simulink model "astron_hw_test_au50_64k_8in"  (R2021a)
settings: Solver=VariableStepDiscrete  StartTime=0.0  StopTime=32000  RelTol=1e-3
undefined symbols (not defined in the file): d0, d1, d2, d3, d4, d5, d6, d7, FFT, sr, Wideband_FFT
libraries: xbsIndex_r4 x1247, casper_library_misc x6, xps_library x1
(part 6 of 26)

== system astron_hw_test_au50_64k_8in/bram_in3 ==
  addr : Inport
  data_in : Inport  Port=2
  we : Inport  Port=3
  Terminator : Terminator
  Terminator1 : Terminator
  Terminator2 : Terminator
  astron_hw_test_au50_64k_8in_bram_in3_addr : xbsIndex_r4/Gateway Out  inherit_from_input=off  hdl_port=on  rows=1  columns=1  UseAsDAC=off  DACChannel='1'  interface=None  automatic_assignment=on  address_offset=hex2dec('00')  intf_name=''  intf_description=''  timing_constraint=None  locs_specified=off  LOCs={'A5','B9','A9','C1','A3','G6','E9','A6','A7','A8','B8','B1','B3','D9','B5','B4','B6','C2'}  io_standard={}  block_type=gatewayout
      settings: infoedit="Gateway out block.  Converts Xilinx fixed point inputs into ouputs of type Simulink integer, double, or fixed point.<P><P>Hardware notes:  In hardware these blocks become top level output ports or are discarded, depending on how they are configured."  sginterface={'Nallatech'=>{'xdspkit'=>{'non_memory_mapped_port'=>'uprev_Shared_BRAM_addr'}},'Xilinx'=>{'jtaghwcosim'=>{'non_memory_mapped_port'=>'uprev_Shared_BRAM_addr'},'xdspkit'=>{'non_memory_mapped_port'=>'uprev_Shared_BRAM_addr'}}}  xl_area=[0, 0, 0, 0, 0, 0, 0]
  astron_hw_test_au50_64k_8in_bram_in3_data_in : xbsIndex_r4/Gateway Out  inherit_from_input=off  hdl_port=on  rows=1  columns=1  UseAsDAC=off  DACChannel='1'  interface=None  automatic_assignment=on  address_offset=hex2dec('00')  intf_name=''  intf_description=''  timing_constraint=None  locs_specified=off  LOCs={'B21','B22','A22','B23','B19','C19','A20','A21','A23','B24','A24','A25','E18','D18','C18','B18'}  io_standard={}  block_type=gatewayout
      settings: infoedit="Gateway out block.  Converts Xilinx fixed point inputs into ouputs of type Simulink integer, double, or fixed point.<P><P>Hardware notes:  In hardware these blocks become top level output ports or are discarded, depending on how they are configured."  sginterface={'Nallatech'=>{'xdspkit'=>{'non_memory_mapped_port'=>'uprev_Shared_BRAM_data_in'}},'Xilinx'=>{'jtaghwcosim'=>{'non_memory_mapped_port'=>'uprev_Shared_BRAM_data_in'},'xdspkit'=>{'non_memory_mapped_port'=>'uprev_Shared_BRAM_data_in'}}}  xl_area=[0, 0, 0, 0, 0, 0, 0]
  astron_hw_test_au50_64k_8in_bram_in3_data_out : xbsIndex_r4/Gateway In  gui_display_data_type=Fixed-point  arith_type=Unsigned  n_bits=32  bin_pt=0  preci_type=Single  exp_width=8  frac_width=24  rows=1  columns=1  quantization=Truncate  overflow=Wrap  period=sample_rate  UseAsADC=off  ADCChannel='1'  interface=None  automatic_assignment=on  address_offset=hex2dec('00')  intf_name=''  intf_description=''  default_value=0  timing_constraint=None  locs_specified=off  LOCs={}  io_standard={}  inherit_from_input=off  hdl_port=on  dbl_ovrd=off  block_type=gatewayin
      settings: xl_area=[0, 0, 0, 0, 0, 0, 0]
  astron_hw_test_au50_64k_8in_bram_in3_we : xbsIndex_r4/Gateway Out  inherit_from_input=off  hdl_port=on  rows=1  columns=1  UseAsDAC=off  DACChannel='1'  interface=None  automatic_assignment=on  address_offset=hex2dec('00')  intf_name=''  intf_description=''  timing_constraint=None  locs_specified=off  LOCs={'A14'}  io_standard={}  block_type=gatewayout
      settings: infoedit="Gateway out block.  Converts Xilinx fixed point inputs into ouputs of type Simulink integer, double, or fixed point.<P><P>Hardware notes:  In hardware these blocks become top level output ports or are discarded, depending on how they are configured."  xl_area=[0, 0, 0, 0, 0, 0, 0]
  calc_add : Subsystem  mask{data_width=32, addr_width=13, sample_rate=sample_rate}
      mask prompts: data_width "data width"; addr_width "address width"; sample_rate "sample rate"
  convert_addr : xbsIndex_r4/Convert  gui_display_data_type=Fixed-point  arith_type=Unsigned  n_bits=addr_width  bin_pt=0  float_type=Single  exp_bits=8  fraction_bits=24  quantization=Truncate  overflow=Wrap  en=off  latency=0  pipeline=off  dbl_ovrd=off  block_type=convert
      settings: xl_area=[0, 0, 0, 0, 0, 0, 0]
  convert_din1 : xbsIndex_r4/Convert  gui_display_data_type=Fixed-point  arith_type=Unsigned  n_bits=32  bin_pt=0  float_type=Single  exp_bits=8  fraction_bits=24  quantization=Truncate  overflow=Wrap  en=off  latency=0  pipeline=off  dbl_ovrd=off  block_type=convert
      settings: xl_area=[0, 0, 0, 0, 0, 0, 0]
  convert_we : xbsIndex_r4/Convert  gui_display_data_type=Fixed-point  arith_type=Unsigned  n_bits=1  bin_pt=0  float_type=Single  exp_bits=8  fraction_bits=24  quantization=Truncate  overflow=Wrap  en=off  latency=0  pipeline=off  dbl_ovrd=off  block_type=convert
      settings: xl_area=[0, 0, 0, 0, 0, 0, 0]
  munge_in : Subsystem  AncestorBlock=casper_library_flow_control/munge  mask(munge){divisions=1, div_size=32, order=[0], arith_type_out=Unsigned, bin_pt_out=0}
      mask prompts: divisions "Number of divisions"; div_size "Division size (bits)"; order "Division packing order"; arith_type_out "Output arithmetic type"; bin_pt_out "Output binary point"
      mask help: Splits an input bus into the specified number of divisions and then recombines them in the order specified (most significant division = 0,least = number divisions-1)
      mask init:
      | munge_init(gcb, ...
      |     'divisions', divisions, ...
      |     'div_size', div_size, ...
      |     'order', order, ...
      |     'arith_type_out', arith_type_out, ...
      |     'bin_pt_out', bin_pt_out);
      settings: AttributesFormatString=|
      | split:32
      | join:0
      | Unsigned [32,0]
      mask TypeOptions arith_type_out: Unsigned | Signed  (2's comp) | Floating-point
  munge_out : Subsystem  AncestorBlock=casper_library_flow_control/munge  mask(munge){divisions=1, div_size=32, order=[0], arith_type_out=Signed  (2's comp), bin_pt_out=0}
      mask prompts: divisions "Number of divisions"; div_size "Division size (bits)"; order "Division packing order"; arith_type_out "Output arithmetic type"; bin_pt_out "Output binary point"
      mask help: Splits an input bus into the specified number of divisions and then recombines them in the order specified (most significant division = 0,least = number divisions-1)
      mask init:
      | munge_init(gcb, ...
      |     'divisions', divisions, ...
      |     'div_size', div_size, ...
      |     'order', order, ...
      |     'arith_type_out', arith_type_out, ...
      |     'bin_pt_out', bin_pt_out);
      settings: AttributesFormatString=|
      | split:32
      | join:0
      | Signed  (2's comp) [32,0]
      mask TypeOptions arith_type_out: Unsigned | Signed  (2's comp) | Floating-point
  sim_mem : Subsystem  mask{arith_type=Signed  (2's comp), addr_width=13, data_width=32, data_bin_pt=0, init_vals=[9831  -6047   1111  -1845    944    479  -1311  -4696  10466   2542   1296  -5528   5032   9085  -9007   3196   1045  -2612   4431   2747    701  -2394   4649   7953   7611  -2438    653  -7011   6485  -8623   2524  -5311   5832   3592   -951  -3611   -666  -3316    239  -2256  -3089   3750  -4638   2874   3427  -1997   9115   1935   4089 -10713   4822   2154    279   5735   6850   -832   -441  -4702  -6341    514   3095   -604   4622    495   7543  -1649   5852  -3513  -1426   5023   3080   5056  12109   2829    -89  -1958  -1635   -882   8086   4095   5011  -5808    892  -5959   3390   3640   4469   5622    600  -6979   -735  -1172   3021  -2489    -10 -10282  -7018 -14437   3342    918   4893  -8173   4321   8999   1488  -7407   5292  -5466   8451   -385   1054   1231   9655  -6940  -2235  -3834   2601  -2170   5686  -1603   5214   3496   2809   3538     95  -3789   1812   -759   6389   5558   3719  -1679  -3442   3537   1698  -5286    545    375   2542  -2227   3925   2425   1058   5149   5431   -340    165  -8569   3002  -7189   2921   7702  10866   1098   2719  -6821   5714   2275  -2093  -2390   3583   1045   3029  -5013   2806   4201   -826   4473   1926   3197   2662  -5326   -132  -7657   6141  -3966   1085   4296   2972     60   2145   3502    -45   -413   -959  -8354   5105  -1323 -10075  -3461   4303  -2691   2921   2691   2602  -4447   2141   8240   2358  -1447   4984  -4375   7550  -4944  -4384  -9436   2974  -2464   4849  -3601    -81  -2469  11803   3804    -66  -9192   8238  -2284   6592  -4265   3099  -6350   3474  -1622  -2254  -3545  -4155  -5390   4483   1566  -1045  -8853   -741  -3638   4152   9605    557  -9120   -787  -1927    850  -1036  10537  -4090   3719  -3434  12818  -2443   4345  -2115  -2682   1417   2999   -762  -3818   8830   5004    283   4847    593   7089   5204  -3732  -9948   7734  -8598  -1826  -6373   2929  -6636   8898  -6733   2805   -596  -5987  -4944   7847    510   1205   3500    382   -598    -97  -4652   1154   -953   3535  -2441   7111  -9693   3713  -3212   1794  -5432    301   -702  -1188    492   -793   2941  -4045   -111  -4155  -3060    -51   5492   3268  -4313  -1345  -7136   2901   1051   5939  -3694   8840   2262   -403  -5610   4756  -7788   6039  -3389  -2091  -2286   3817  -4211   8586  -2541  -3705   1884  -3454   -887  -1307   3129  -6280  -4930   8462    603   5506   5738   -144  -5426  -3299  -1591  -6466  -5500   1847  -5378  -1050   7636    689   7195  -1804    850  -4646    703   6319   -691    253   1289   2303  -5210    -98  -5311   8003   5818  -1783    215   8450  -6400   6456  -5666   2753  -6368   2782  -2959  -1937  -3602   -487   5704   5510   1630   2078  -4597   -948  -6721   4817   2330   6877  -1355   1003  -5600   6903   -879    735  -2590  -2126  -1524   2499  -3501   2332  -5911  -2813  -6443   3256  -1249   2184  -4319   2119  -4953   1788   2230   1784  -2352   2383  -2460   -447  -1967   4260   6169   3182  -1023   1018  -1144    406  -5783   5254  -1791   4638  -1833   1731   3018   9039   1357   -962  -3203    806   1286   1434  -2502   5136   -596   2284   1981   2855   -878   -922   -572   2006  -2235  -2959  -5549   4506  -1686   -573   3012  10319  -3694   4335   -511   7943     82   1077  -5232    597  -8641   7231   9600   1123   3237   2347   1991   8087   -763   3952   1484   5065  -1510   5204   3758   3772  -5195  -1555   1894   5991  -2296   2287 -10361  -4481    696   6723  -2738  -6323  -1676  -2645  -4943   7126  -4801    931  -1829   -664   5356   1132  -2373  -2661  -2493   7901    563   -185  -6042   2893  -4373    839  -9450  -1901  -2670   3477  -4903   2623  -6346    573  -2725   2788  -8561  -5178   2433   4219  -2783    -88    688  -6513  -1114  -8548   3020   -325  -4145  -1442   3024  -1441  -1858   3081   -849   4683  -8922   5722   5566   4522  -2714   3565  -4945  -2353  -6535   1476  -3042  -2745   4685   4306   1166    144  -7604   1129   -849   3398  -4810  -5030  -2266   5124   -925   2510  -1880    236 ...(+53345 chars)], sample_rate=1, csp_latency=1}
      mask prompts: arith_type "Output Data Type"; addr_width "Address width"; data_width "Data width"; data_bin_pt "Data Binary Point"; init_vals "Initial values"; sample_rate "Sample rate"; csp_latency "Latency"
      mask init:
      | % set_param([gcb, '/data_to_xilinx'], 'arith_type', arith_type)
      | % set_param([gcb, '/data_to_xilinx'], 'n_bits', get_param(gcb, 'data_width'))
      mask TypeOptions arith_type: Unsigned | Signed  (2's comp)
      mask TypeOptions data_width: 8 | 16 | 32 | 64 | 128
  data_out : Outport  VectorParamsAs1DForOutWhenUnconnected=off
  wires:
  munge_out/1(dout) -> data_out/1
  sim_mem/1(data_out) -> astron_hw_test_au50_64k_8in_bram_in3_data_out/1
  astron_hw_test_au50_64k_8in_bram_in3_data_out/1 -> munge_out/1(din)
  convert_addr/1 -> astron_hw_test_au50_64k_8in_bram_in3_addr/1
  convert_din1/1 -> astron_hw_test_au50_64k_8in_bram_in3_data_in/1
  data_in/1 -> munge_in/1(din)
  calc_add/1(out) -> convert_addr/1
  astron_hw_test_au50_64k_8in_bram_in3_we/1 -> Terminator2/1
  astron_hw_test_au50_64k_8in_bram_in3_data_in/1 -> Terminator1/1
  astron_hw_test_au50_64k_8in_bram_in3_addr/1 -> Terminator/1
  convert_we/1 -> astron_hw_test_au50_64k_8in_bram_in3_we/1
  addr/1 -> sim_mem/1(addr), calc_add/1(in)
  we/1 -> sim_mem/3(we), convert_we/1
  munge_in/1(dout) -> sim_mem/2(data), convert_din1/1
